simulink model "SoftABS"  (Simulink 7.5)
settings: Solver=ode45  StartTime=0.0  StopTime=inf  RelTol=1e-3
PreLoadFcn:
  | SoftABS_params
undefined symbols (not defined in the file): f_ax, f_slip, sko, sku, T_F_Pres_Free, T_F_Pres_Keep, T_F_Pres_Reduce
libraries: CarMaker4SL x13, simulink x1
(part 1 of 2)
settings Model: Creator=fh  LastModifiedBy=ml  ExtModeAutoUpdateStatusClock=off
settings DataIOCC: SignalLoggingName=sigsOut
settings OptimizationCC: BooleanDataType=off  InitFltsAndDblsToZero=on
settings DebuggingCC: SaveWithParameterizedLinksMsg=none  SignalResolutionControl=TryResolveAllWithWarning  SolverPrmCheckMsg=none  MultiTaskDSMMsg=warning  MultiTaskCondExecSysMsg=none
settings HardwareCC: TargetUnknown=on
settings RTWCC: IncludeERTFirstTime=on
settings CodeAppCC: MaxIdLength=63
settings GRTTargetCC: TargetFcnLib=ansi_tfl_tmw.mat

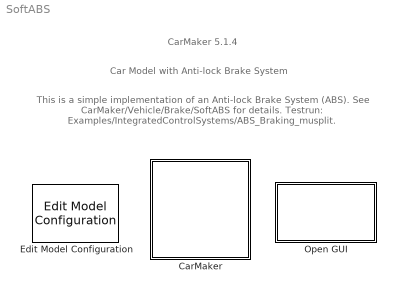
== system SoftABS ==
  note: Car Model with Anti-lock Brake System
  note: CarMaker 5.1.4
  note: This is a simple implementation of an Anti-lock Brake System (ABS).
      | See CarMaker/Vehicle/Brake/SoftABS for details.
      | Testrun: Examples/IntegratedControlSystems/ABS_Braking_musplit.
  CarMaker : Subsystem  TreatAsAtomicUnit=on
      mask Display: image(imread('CarMaker4SLss.bmp'));
  Edit Model Configuration : CarMaker4SL/Edit Model Configuration
  Open GUI : Subsystem  LoadFcn=if ~length(which('cmcmd')), cmenv; end
      settings: OpenFcn=cmblockmagic('gui_fix_display'); CM_Simulink
      mask Display: image(imread('CarMakerGUI.bmp'));

== system SoftABS/CarMaker ==
  CM_FIRST : Subsystem
  CM_LAST : Subsystem
  DrivMan : Subsystem
  Ground : Ground
  Terminator : Terminator
  Vehicle : Subsystem
  VehicleControl : Subsystem
  wires:
  DrivMan/2(DrivMan.Out) -> VehicleControl/2(DrivMan.In)
  DrivMan/1(Sync_Out) -> VehicleControl/1(Sync_In)
  CM_FIRST/2(Env.Misc) -> DrivMan/2(Env.Misc)
  CM_FIRST/1(Sync_Out) -> DrivMan/1(Sync_In)
  CM_LAST/1(Sync_Out) -> Terminator/1
  Ground/1 -> CM_FIRST/1(Sync_In)
  Vehicle/1(Sync_Out) -> CM_LAST/1(Sync_In)
  VehicleControl/1(Sync_Out) -> Vehicle/1(Sync_In)
  VehicleControl/3(VhclCtrl.Steering) -> Vehicle/3(VhclCtrl.Steering)
  VehicleControl/4(Vhcl.Wheel.In) -> Vehicle/4(Vhcl.Wheel.In)
  VehicleControl/5(Vhcl.Misc) -> Vehicle/5(Vhcl.Misc)
  VehicleControl/6(VhclCtrl.Brake) -> Vehicle/6(VhclCtrl.Brake)
  VehicleControl/7(VhclCtrl.PT) -> Vehicle/7(VhclCtrl.PT)
  VehicleControl/2(Vhcl.Model.Source) -> Vehicle/2(Vhcl.Model.Source)

== system SoftABS/Open GUI ==
  S-Function : S-Function  FunctionName=cm_gui  EnableBusSupport=off

== system SoftABS/CarMaker/CM_FIRST ==
  Sync_In : Inport  OutDataType=sfix(16)  OutScaling=2^0
  Bus Creator1 : BusCreator  Inputs=9
  Demux : Demux  Outputs=9
  Environment : S-Function  FunctionName=CM_Sfun  Parameters='Environment'  EnableBusSupport=off
  IoIn : S-Function  FunctionName=CM_Sfun  Parameters='IoIn'  EnableBusSupport=off
  Sync_Out : Outport  OutDataType=sfix(16)  OutScaling=2^0
  Env.Misc : Outport  Port=2  OutDataType=sfix(16)  OutScaling=2^0
  wires:
  Demux/9 -> Bus Creator1/9  "Env WindVel_tot z"
  Demux/8 -> Bus Creator1/8  "Env WindVel_tot y"
  Demux/7 -> Bus Creator1/7  "Env WindVel_tot x"
  Demux/6 -> Bus Creator1/6  "Env SolarRadiation"
  Demux/5 -> Bus Creator1/5  "Env Time"
  Sync_In/1 -> IoIn/1
  IoIn/1 -> Environment/1
  Environment/1 -> Sync_Out/1
  Demux/1 -> Bus Creator1/1  "Env Temperature"
  Demux/2 -> Bus Creator1/2  "Env AirDensity"
  Demux/3 -> Bus Creator1/3  "Env AirPressure"
  Demux/4 -> Bus Creator1/4  "Env AirHumidity"
  Environment/2 -> Demux/1
  Bus Creator1/1 -> Env.Misc/1

== system SoftABS/CarMaker/CM_LAST ==
  Sync_In : Inport  OutDataType=sfix(16)  OutScaling=2^0
  CM_User : S-Function  FunctionName=CM_Sfun  Parameters='CM_User'  EnableBusSupport=off
  IoOut : S-Function  FunctionName=CM_Sfun  Parameters='IoOut'  EnableBusSupport=off
  Sync_Out : Outport  OutDataType=sfix(16)  OutScaling=2^0
  wires:
  IoOut/1 -> Sync_Out/1
  CM_User/1 -> IoOut/1
  Sync_In/1 -> CM_User/1

== system SoftABS/CarMaker/DrivMan ==
  note: There's rarely a reason to override DrivMan signals.
      | Use the VehicleControl interface for this purpose.
  Sync_In : Inport  OutDataType=sfix(16)  OutScaling=2^0
  Env.Misc : Inport  Port=2  OutDataType=sfix(16)  OutScaling=2^0
  BusCreator : BusCreator  Inputs=17
  Demux : Demux  Outputs=17
  DrivMan : S-Function  FunctionName=CM_Sfun  Parameters='DrivMan'  EnableBusSupport=off
  Sync_Out : Outport  OutDataType=sfix(16)  OutScaling=2^0
  DrivMan.Out : Outport  Port=2  OutDataType=sfix(16)  OutScaling=2^0
  wires:
  DrivMan/2 -> Demux/1
  BusCreator/1 -> DrivMan.Out/1
  DrivMan/1 -> Sync_Out/1
  Sync_In/1 -> DrivMan/1
  Env.Misc/1 -> DrivMan/2
  Demux/1 -> BusCreator/1  "DrivMan SST"
  Demux/2 -> BusCreator/2  "DrivMan Key"
  Demux/3 -> BusCreator/3  "DrivMan UserSignal0"
  Demux/4 -> BusCreator/4  "DrivMan UserSignal1"
  Demux/5 -> BusCreator/5  "DrivMan UserSignal2"
  Demux/6 -> BusCreator/6  "DrivMan UserSignal3"
  Demux/7 -> BusCreator/7  "DrivMan UserSignal4"
  Demux/8 -> BusCreator/8  "DrivMan SelectorCtrl"
  Demux/9 -> BusCreator/9  "DrivMan GearNo"
  Demux/10 -> BusCreator/10  "DrivMan Brake"
  Demux/11 -> BusCreator/11  "DrivMan BrakePark"
  Demux/12 -> BusCreator/12  "DrivMan Clutch"
  Demux/13 -> BusCreator/13  "DrivMan Gas"
  Demux/14 -> BusCreator/14  "DrivMan Steering Ang"
  Demux/15 -> BusCreator/15  "DrivMan Steering AngVel"
  Demux/16 -> BusCreator/16  "DrivMan Steering AngAcc"
  Demux/17 -> BusCreator/17  "DrivMan Steering Trq"

== system SoftABS/CarMaker/Vehicle ==
  Sync_In : Inport  OutDataType=sfix(16)  OutScaling=2^0
  Vhcl.Model.Source : Inport  Port=2  OutDataType=sfix(16)  OutScaling=2^0
  VhclCtrl.Steering : Inport  Port=3  OutDataType=sfix(16)  OutScaling=2^0
  Vhcl.Wheel.In : Inport  Port=4  OutDataType=sfix(16)  OutScaling=2^0
  Vhcl.Misc : Inport  Port=5  OutDataType=sfix(16)  OutScaling=2^0
  VhclCtrl.Brake : Inport  Port=6  OutDataType=sfix(16)  OutScaling=2^0
  VhclCtrl.PT : Inport  Port=7  OutDataType=sfix(16)  OutScaling=2^0
  Brake : Subsystem
  CarAndTrailer : Subsystem
  PowerTrain : Subsystem
  Stop Simulation : Stop
  VehicleSource_BuiltIn : simulink/Logic and Bit Operations/Compare To Constant  SystemSampleTime=-1  relop=~=  const=1  LogicOutDataTypeMode=boolean  ZeroCross=off
  Sync_Out : Outport  OutDataType=sfix(16)  OutScaling=2^0
  wires:
  Vhcl.Model.Source/1 -> VehicleSource_BuiltIn/1
  Sync_In/1 -> CarAndTrailer/1(Sync_In)
  VhclCtrl.Steering/1 -> CarAndTrailer/2(VhclCtrl.Steering)
  Vhcl.Wheel.In/1 -> CarAndTrailer/3(Vhcl.Wheel.In)
  Vhcl.Misc/1 -> CarAndTrailer/4(Vhcl.Misc)
  PowerTrain/1(Sync_Out) -> Sync_Out/1
  VhclCtrl.Brake/1 -> Brake/3(VhclCtrl.Brake)
  CarAndTrailer/2(Brake.IF.In) -> Brake/2(Brake.IF.In)
  CarAndTrailer/1(Sync_Out) -> Brake/1(Sync_In)
  VhclCtrl.PT/1 -> PowerTrain/3(VhclCtrl.PT)
  VehicleSource_BuiltIn/1 -> Stop Simulation/1
  Brake/1(Sync_Out) -> PowerTrain/1(Sync_In)
  Brake/2(Vhcl.Wheel.PT) -> PowerTrain/2(Vhcl.Wheel.PT)

== system SoftABS/CarMaker/VehicleControl ==
  note: <Your model here>
  note: When implementing a vehicle control model,
      | be sure to add '-disablevehiclecontrol' to the command line arguments
      | in the CarMaker Model Configuration block.
      | Otherwise your model will possibly not see the original DrivMan signals
      | on its inputs, but those of a currently activated C-coded vehicle control model instead.
  Sync_In : Inport  OutDataType=sfix(16)  OutScaling=2^0
  DrivMan.In : Inport  Port=2  OutDataType=sfix(16)  OutScaling=2^0
  Bus Creator2 : BusCreator  Inputs=2
  CreateBus Vhcl.Misc : Subsystem
  CreateBus Vhcl.Wheel.In : Subsystem
  CreateBus VhclCtrl : Subsystem
  CreateBus VhclCtrl.PT : Subsystem
  CreateBus VhclCtrl.Steering : Subsystem
  Demux2 : Demux  Outputs=2
  VehicleControl : S-Function  FunctionName=CM_Sfun  Parameters='VehicleControl'  EnableBusSupport=off
  VehicleControlUpd : S-Function  FunctionName=CM_Sfun  Parameters='VehicleControlUpd'  EnableBusSupport=off
  Sync_Out : Outport  OutDataType=sfix(16)  OutScaling=2^0
  Vhcl.Model.Source : Outport  Port=2  OutDataType=sfix(16)  OutScaling=2^0
  VhclCtrl.Steering : Outport  Port=3  OutDataType=sfix(16)  OutScaling=2^0
  Vhcl.Wheel.In : Outport  Port=4  OutDataType=sfix(16)  OutScaling=2^0
  Vhcl.Misc : Outport  Port=5  OutDataType=sfix(16)  OutScaling=2^0
  VhclCtrl.Brake : Outport  Port=6  OutDataType=sfix(16)  OutScaling=2^0
  VhclCtrl.PT : Outport  Port=7  OutDataType=sfix(16)  OutScaling=2^0
  wires:
  CreateBus VhclCtrl/1(Out) -> VehicleControlUpd/2
  VehicleControl/2 -> CreateBus VhclCtrl/1(In)
  VehicleControlUpd/2 -> Vhcl.Model.Source/1
  VehicleControlUpd/4 -> CreateBus Vhcl.Wheel.In/1(In1)
  VehicleControlUpd/5 -> CreateBus Vhcl.Misc/1(In1)
  VehicleControlUpd/6 -> Demux2/1
  VehicleControlUpd/7 -> CreateBus VhclCtrl.PT/1(In1)
  VehicleControlUpd/3 -> CreateBus VhclCtrl.Steering/1(In1)
  CreateBus Vhcl.Misc/1(Out1) -> Vhcl.Misc/1
  CreateBus Vhcl.Wheel.In/1(Out1) -> Vhcl.Wheel.In/1
  DrivMan.In/1 -> VehicleControl/2
  VehicleControl/1 -> VehicleControlUpd/1
  Sync_In/1 -> VehicleControl/1
  CreateBus VhclCtrl.PT/1(Out1) -> VhclCtrl.PT/1
  Bus Creator2/1 -> VhclCtrl.Brake/1
  CreateBus VhclCtrl.Steering/1(Out1) -> VhclCtrl.Steering/1
  VehicleControlUpd/1 -> Sync_Out/1
  Demux2/2 -> Bus Creator2/2  "VhclCtrl BrakePark"
  Demux2/1 -> Bus Creator2/1  "VhclCtrl Brake"

== system SoftABS/CarMaker/Vehicle/Brake ==
  note: When replacing the entire braking system,
      | be sure to add '-disablebrake' to the command line arguments
      | in the CarMaker Model Configuration block.
  Sync_In : Inport  OutDataType=sfix(16)  OutScaling=2^0
  Brake.IF.In : Inport  Port=2  OutDataType=sfix(16)  OutScaling=2^0
  VhclCtrl.Brake : Inport  Port=3  OutDataType=sfix(16)  OutScaling=2^0
  Brake : S-Function  FunctionName=CM_Sfun  Parameters='Brake'  EnableBusSupport=off
  BrakeUpd : S-Function  FunctionName=CM_Sfun  Parameters='BrakeUpd'  EnableBusSupport=off
  BusCreator : BusCreator  Inputs=12
  CreateBus Vhcl.Wheel.PT : Subsystem
  Demux : Demux  Outputs=12
  SoftABS : Subsystem
  Sync_Out : Outport  OutDataType=sfix(16)  OutScaling=2^0
  Vhcl.Wheel.PT : Outport  Port=2  OutDataType=sfix(16)  OutScaling=2^0
  wires:
  Brake/1 -> BrakeUpd/1  "Sync"
  Brake.IF.In/1 -> Brake/2
  VhclCtrl.Brake/1 -> Brake/3
  Brake/2 -> Demux/1
  Sync_In/1 -> Brake/1
  BusCreator/1 -> SoftABS/1(Brake.In)
  SoftABS/1(Brake.Out) -> BrakeUpd/2
  Demux/12 -> BusCreator/12  "Brake IF Trq_Reg_trg RR"
  Demux/11 -> BusCreator/11  "Brake IF Trq_Reg_trg RL"
  Demux/10 -> BusCreator/10  "Brake IF Trq_Reg_trg FR"
  Demux/9 -> BusCreator/9  "Brake IF Trq_Reg_trg FL"
  Demux/8 -> BusCreator/8  "Brake IF Trq_PB RR"
  Demux/7 -> BusCreator/7  "Brake IF Trq_PB RL"
  Demux/6 -> BusCreator/6  "Brake IF Trq_PB FR"
  Demux/5 -> BusCreator/5  "Brake IF Trq_PB FL"
  Demux/4 -> BusCreator/4  "Brake IF Trq_WB RR"
  Demux/3 -> BusCreator/3  "Brake IF Trq_WB RL"
  Demux/2 -> BusCreator/2  "Brake IF Trq_WB FR"
  Demux/1 -> BusCreator/1  "Brake IF Trq_WB FL"
  BrakeUpd/1 -> Sync_Out/1
  BrakeUpd/2 -> CreateBus Vhcl.Wheel.PT/1(In)
  CreateBus Vhcl.Wheel.PT/1(Out) -> Vhcl.Wheel.PT/1

== system SoftABS/CarMaker/Vehicle/CarAndTrailer ==
  Sync_In : Inport  OutDataType=sfix(16)  OutScaling=2^0
  VhclCtrl.Steering : Inport  Port=2  OutDataType=sfix(16)  OutScaling=2^0
  Vhcl.Wheel.In : Inport  Port=3  OutDataType=sfix(16)  OutScaling=2^0
  Vhcl.Misc : Inport  Port=4  OutDataType=sfix(16)  OutScaling=2^0
  CarAndTrailerUpd : Subsystem
  Forces : Subsystem
  Ground : Ground
  Kinematics : Subsystem
  Kinetics : Subsystem
  Steering : Subsystem
  Terminator : Terminator
  Terminator1 : Terminator
  Trailer : Subsystem
  Sync_Out : Outport  OutDataType=sfix(16)  OutScaling=2^0
  Brake.IF.In : Outport  Port=2  OutDataType=sfix(16)  OutScaling=2^0
  wires:
  Kinematics/9(lBuf) -> Forces/9(lBuf)
  Forces/12(FBuf) -> Kinetics/12(FBuf)
  Kinematics/8(lStabi) -> Forces/8(lStabi)
  Kinematics/1(Sync_Out) -> Forces/1(Sync_In)
  Kinematics/2(TireFL_In) -> Forces/2(TireFL_In)
  Kinematics/3(TireFR_In) -> Forces/3(TireFR_In)
  Kinematics/4(TireRL_In) -> Forces/4(TireRL_In)
  Kinematics/5(TireRR_In) -> Forces/5(TireRR_In)
  Forces/1(Sync_Out) -> Kinetics/1(Sync_In)
  Forces/3(Car.Aero) -> Kinetics/3(Car.Aero)
  Kinematics/7(vDamp) -> Forces/7(vDamp)
  Kinematics/6(lSpring) -> Forces/6(lSpring)
  Forces/2(Car.Virtual) -> Kinetics/2(Car.Virtual)
  Forces/4(Car.Load) -> Kinetics/4(Car.Load)
  Forces/5(TireFL_Out) -> Kinetics/5(TireFL.Out)
  Forces/6(TireFR_Out) -> Kinetics/6(TireFR.Out)
  Forces/7(TireRL_Out) -> Kinetics/7(TireRL.Out)
  Forces/8(TireRR_Out) -> Kinetics/8(TireRR.Out)
  Forces/9(FSpring) -> Kinetics/9(FSpring)
  Forces/10(FDamp) -> Kinetics/10(FDamp)
  Forces/11(FStabi) -> Kinetics/11(FStabi)
  Ground/1 -> CarAndTrailerUpd/10(Vhcl.Fr1A)
  Kinetics/1(Sync_Out) -> Trailer/1(Sync_In)
  Steering/1(Sync_Out) -> Kinematics/1(Sync_In)
  Sync_In/1 -> Steering/1(Sync_In)
  VhclCtrl.Steering/1 -> Steering/2(VhclCtrl.Steering)
  Kinetics/2(Trailer.Load) -> Trailer/2(Trailer.Load)
  Kinetics/3(Car.Hitch) -> Trailer/3(Car.Hitch)
  Kinetics/4(Car.Fr1) -> Trailer/4(Car.Fr1)
  Steering/2(Steer.IF) -> Kinematics/2(Steer.IF)
  Kinetics/5(Car.Trq_T2W) -> Trailer/5(Car.Trq_T2W)
  Kinetics/6(WheelCarrier.Misc) -> Trailer/6(WheelCarrier.Misc)
  Vhcl.Wheel.In/1 -> Terminator/1
  Vhcl.Misc/1 -> Terminator1/1
  CarAndTrailerUpd/1(Sync_Out) -> Sync_Out/1
  CarAndTrailerUpd/2(Brake.IF.In) -> Brake.IF.In/1
  Trailer/1(Sync_Out) -> CarAndTrailerUpd/1(Sync_In)
  Trailer/2(Vhcl.Steering) -> CarAndTrailerUpd/2(Vhcl.Steering)
  Trailer/3(Vhcl.Motion) -> CarAndTrailerUpd/3(Vhcl.Motion)
  Trailer/4(Vhcl.PoI) -> CarAndTrailerUpd/4(Vhcl.PoI)
  Trailer/5(Vhcl.Wheel.FL) -> CarAndTrailerUpd/5(Vhcl.Wheel.FL)
  Trailer/6(Vhcl.Wheel.FR) -> CarAndTrailerUpd/6(Vhcl.Wheel.FR)
  Trailer/7(Vhcl.Wheel.RL) -> CarAndTrailerUpd/7(Vhcl.Wheel.RL)
  Trailer/8(Vhcl.Wheel.RR) -> CarAndTrailerUpd/8(Vhcl.Wheel.RR)
  Trailer/9(Car.Hitch.FrcTrq) -> CarAndTrailerUpd/9(Car.Hitch.FrcTrq)

== system SoftABS/CarMaker/Vehicle/PowerTrain ==
  note: <Your model here>
  note: When replacing the entire powertrain,
      | be sure to add '-disablepowertrain' to the command line arguments
      | in the CarMaker Model Configuration block.
  Sync_In : Inport  OutDataType=sfix(16)  OutScaling=2^0
  Vhcl.Wheel.PT : Inport  Port=2  OutDataType=sfix(16)  OutScaling=2^0
  VhclCtrl.PT : Inport  Port=3  OutDataType=sfix(16)  OutScaling=2^0
  BusCreator : BusCreator  Inputs=40
  Demux : Demux  Outputs=40
  PowerTrain : S-Function  FunctionName=CM_Sfun  Parameters='PowerTrain'  EnableBusSupport=off
  PowerTrainUpd : S-Function  FunctionName=CM_Sfun  Parameters='PowerTrainUpd'  EnableBusSupport=off
  Sync_Out : Outport  OutDataType=sfix(16)  OutScaling=2^0
  wires:
  Vhcl.Wheel.PT/1 -> PowerTrain/2
  VhclCtrl.PT/1 -> PowerTrain/3
  Demux/40 -> BusCreator/40  "PT IF WRR Trq_BrakeReg_max"
  Demux/39 -> BusCreator/39  "PT IF WRR Trq_BrakeReg"
  Demux/38 -> BusCreator/38  "PT IF WRR Trq_Supp2WC"
  Demux/37 -> BusCreator/37  "PT IF WRR Trq_Drive"
  Demux/36 -> BusCreator/36  "PT IF WRR Trq_B2W"
  Demux/35 -> BusCreator/35  "PT IF WRR rotv"
  Demux/34 -> BusCreator/34  "PT IF WRR rot"
  Demux/33 -> BusCreator/33  "PT IF WRL Trq_BrakeReg_max"
  Demux/32 -> BusCreator/32  "PT IF WRL Trq_BrakeReg"
  Demux/31 -> BusCreator/31  "PT IF WRL Trq_Supp2WC"
  Demux/30 -> BusCreator/30  "PT IF WRL Trq_Drive"
  Demux/29 -> BusCreator/29  "PT IF WRL Trq_B2W"
  Demux/28 -> BusCreator/28  "PT IF WRL rotv"
  Demux/27 -> BusCreator/27  "PT IF WRL rot"
  Demux/26 -> BusCreator/26  "PT IF WFR Trq_BrakeReg_max"
  Demux/25 -> BusCreator/25  "PT IF WFR Trq_BrakeReg"
  Demux/24 -> BusCreator/24  "PT IF WFR Trq_Supp2WC"
  Demux/23 -> BusCreator/23  "PT IF WFR Trq_Drive"
  Demux/22 -> BusCreator/22  "PT IF WFR Trq_B2W"
  Demux/21 -> BusCreator/21  "PT IF WFR rotv"
  Demux/20 -> BusCreator/20  "PT IF WFR rot"
  Demux/19 -> BusCreator/19  "PT IF WFL Trq_BrakeReg_max"
  Demux/18 -> BusCreator/18  "PT IF WFL Trq_BrakeReg"
  Demux/17 -> BusCreator/17  "PT IF WFL Trq_Supp2WC"
  Demux/16 -> BusCreator/16  "PT IF WFL Trq_Drive"
  Demux/15 -> BusCreator/15  "PT IF WFL Trq_B2W"
  Demux/14 -> BusCreator/14  "PT IF WFL rotv"
  Demux/13 -> BusCreator/13  "PT IF WFL rot"
  Demux/12 -> BusCreator/12  "PT IF DL_iDiff_mean"
  Demux/11 -> BusCreator/11  "PT IF Trq_Supp2BdyEng y"
  Demux/10 -> BusCreator/10  "PT IF Trq_Supp2BdyEng x"
  Demux/9 -> BusCreator/9  "PT IF Trq_Supp2Bdy1 z"
  Demux/8 -> BusCreator/8  "PT IF Trq_Supp2Bdy1 y"
  Demux/7 -> BusCreator/7  "PT IF Trq_Supp2Bdy1 x"
  Demux/6 -> BusCreator/6  "PT IF Engine_Trq (EngineControl)"
  Demux/5 -> BusCreator/5  "PT IF Engine_rotv"
  Demux/4 -> BusCreator/4  "PT IF GearNo"
  Demux/3 -> BusCreator/3  "PT IF OperationError"
  Demux/2 -> BusCreator/2  "PT IF OperationState"
  Demux/1 -> BusCreator/1  "PT IF Ignition"
  BusCreator/1 -> PowerTrainUpd/2
  PowerTrain/1 -> PowerTrainUpd/1  "Sync"
  PowerTrainUpd/1 -> Sync_Out/1
  PowerTrain/2 -> Demux/1
  Sync_In/1 -> PowerTrain/1

== system SoftABS/CarMaker/VehicleControl/CreateBus Vhcl.Misc ==
  In1 : Inport  OutDataType=sfix(16)  OutScaling=2^0
  Bus Creator5 : BusCreator  Inputs=11
  Demux5 : Demux  Outputs=11
  Out1 : Outport  OutDataType=sfix(16)  OutScaling=2^0
  wires:
  Demux5/11 -> Bus Creator5/11  "Vhcl Wind_vel_0 z"
  Demux5/10 -> Bus Creator5/10  "Vhcl Wind_vel_0 y"
  Demux5/9 -> Bus Creator5/9  "Vhcl Wind_vel_0 x"
  Demux5/8 -> Bus Creator5/8  "Vhcl DL2BdyEng y"
  Demux5/7 -> Bus Creator5/7  "Vhcl DL2BdyEng x"
  Demux5/6 -> Bus Creator5/6  "Vhcl TrqDL2Bdy1B z"
  Demux5/5 -> Bus Creator5/5  "Vhcl TrqDL2Bdy1B y"
  Demux5/4 -> Bus Creator5/4  "Vhcl TrqDL2Bdy1B x"
  Demux5/3 -> Bus Creator5/3  "Vhcl Trq_DL2Bdy1 z"
  In1/1 -> Demux5/1
  Bus Creator5/1 -> Out1/1
  Demux5/2 -> Bus Creator5/2  "Vhcl Trq_DL2Bdy1 y"
  Demux5/1 -> Bus Creator5/1  "Vhcl Trq_DL2Bdy1 x"

== system SoftABS/CarMaker/VehicleControl/CreateBus Vhcl.Wheel.In ==
  In1 : Inport  OutDataType=sfix(16)  OutScaling=2^0
  Bus Creator1 : BusCreator  Inputs=12
  Demux1 : Demux  Outputs=12
  Out1 : Outport  OutDataType=sfix(16)  OutScaling=2^0
  wires:
  Demux1/12 -> Bus Creator1/12  "Vhcl Wheel RR rotv"
  Demux1/11 -> Bus Creator1/11  "Vhcl Wheel RR Trq_DL2WC"
  Demux1/10 -> Bus Creator1/10  "Vhcl Wheel RR Trq_B2WC"
  Demux1/9 -> Bus Creator1/9  "Vhcl Wheel RL rotv"
  Demux1/8 -> Bus Creator1/8  "Vhcl Wheel RL Trq_DL2WC"
  Demux1/7 -> Bus Creator1/7  "Vhcl Wheel RL Trq_B2WC"
  Demux1/6 -> Bus Creator1/6  "Vhcl Wheel FR rotv"
  Demux1/5 -> Bus Creator1/5  "Vhcl Wheel FR Trq_DL2WC"
  Demux1/4 -> Bus Creator1/4  "Vhcl Wheel FR Trq_B2WC"
  Demux1/3 -> Bus Creator1/3  "Vhcl Wheel FL rotv"
  In1/1 -> Demux1/1
  Bus Creator1/1 -> Out1/1
  Demux1/2 -> Bus Creator1/2  "Vhcl Wheel FL Trq_DL2WC"
  Demux1/1 -> Bus Creator1/1  "Vhcl Wheel FL Trq_B2WC"

== system SoftABS/CarMaker/VehicleControl/CreateBus VhclCtrl ==
  In : Inport
  BusCreator : BusCreator  Inputs=29
  Demux : Demux  Outputs=29
  Out : Outport
  wires:
  In/1 -> Demux/1
  BusCreator/1 -> Out/1
  Demux/1 -> BusCreator/1  "VhclCtrl SST"
  Demux/2 -> BusCreator/2  "VhclCtrl Key"
  Demux/3 -> BusCreator/3  "VhclCtrl UserSignal0"
  Demux/4 -> BusCreator/4  "VhclCtrl UserSignal1"
  Demux/5 -> BusCreator/5  "VhclCtrl UserSignal2"
  Demux/6 -> BusCreator/6  "VhclCtrl UserSignal3"
  Demux/7 -> BusCreator/7  "VhclCtrl UserSignal4"
  Demux/8 -> BusCreator/8  "VhclCtrl GearNo"
  Demux/9 -> BusCreator/9  "VhclCtrl SelectorCtrl"
  Demux/10 -> BusCreator/10  "VhclCtrl Brake"
  Demux/11 -> BusCreator/11  "VhclCtrl BrakePark"
  Demux/12 -> BusCreator/12  "VhclCtrl Clutch"
  Demux/13 -> BusCreator/13  "VhclCtrl Gas"
  Demux/14 -> BusCreator/14  "VhclCtrl Steering Ang"
  Demux/15 -> BusCreator/15  "VhclCtrl Steering AngVel"
  Demux/16 -> BusCreator/16  "VhclCtrl Steering AngAcc"
  Demux/17 -> BusCreator/17  "VhclCtrl Steering Trq"
  Demux/18 -> BusCreator/18  "VhclCtrl Lights LowBeam"
  Demux/19 -> BusCreator/19  "VhclCtrl Lights HighBeam"
  Demux/20 -> BusCreator/20  "VhclCtrl Lights Daytime"
  Demux/21 -> BusCreator/21  "VhclCtrl Lights ParkL"
  Demux/22 -> BusCreator/22  "VhclCtrl Lights ParkR"
  Demux/23 -> BusCreator/23  "VhclCtrl Lights IndL"
  Demux/24 -> BusCreator/24  "VhclCtrl Lights IndR"
  Demux/25 -> BusCreator/25  "VhclCtrl Lights FogFrontL"
  Demux/26 -> BusCreator/26  "VhclCtrl Lights FogFrontR"
  Demux/27 -> BusCreator/27  "VhclCtrl Lights FogRear"
  Demux/28 -> BusCreator/28  "VhclCtrl Lights Brake"
  Demux/29 -> BusCreator/29  "VhclCtrl Lights Reverse"

== system SoftABS/CarMaker/VehicleControl/CreateBus VhclCtrl.PT ==
  In1 : Inport
  BusCreator : BusCreator  Inputs=11
  Demux : Demux  Outputs=11
  Out1 : Outport
  wires:
  In1/1 -> Demux/1
  BusCreator/1 -> Out1/1
  Demux/1 -> BusCreator/1  "VhclCtrl SST"
  Demux/2 -> BusCreator/2  "VhclCtrl Key"
  Demux/3 -> BusCreator/3  "VhclCtrl UserSignal0"
  Demux/4 -> BusCreator/4  "VhclCtrl UserSignal1"
  Demux/5 -> BusCreator/5  "VhclCtrl UserSignal2"
  Demux/6 -> BusCreator/6  "VhclCtrl UserSignal3"
  Demux/7 -> BusCreator/7  "VhclCtrl UserSignal4"
  Demux/8 -> BusCreator/8  "VhclCtrl GearNo"
  Demux/9 -> BusCreator/9  "VhclCtrl SelectorCtrl"
  Demux/10 -> BusCreator/10  "VhclCtrl Clutch"
  Demux/11 -> BusCreator/11  "VhclCtrl Gas"

== system SoftABS/CarMaker/VehicleControl/CreateBus VhclCtrl.Steering ==
  In1 : Inport  OutDataType=sfix(16)  OutScaling=2^0
  Bus Creator : BusCreator  Inputs=5
  Demux : Demux  Outputs=5
  Out1 : Outport  OutDataType=sfix(16)  OutScaling=2^0
  wires:
  In1/1 -> Demux/1
  Bus Creator/1 -> Out1/1
  Demux/1 -> Bus Creator/1  "VhclCtrl Steering Ang"
  Demux/5 -> Bus Creator/5  "VhclCtrl Steering ByTrq"
  Demux/3 -> Bus Creator/3  "VhclCtrl Steering AngAcc"
  Demux/2 -> Bus Creator/2  "VhclCtrl Steering AngVel"
  Demux/4 -> Bus Creator/4  "VhclCtrl Steering Trq"

== system SoftABS/CarMaker/Vehicle/Brake/CreateBus Vhcl.Wheel.PT ==
  In : Inport
  BusCreator : BusCreator  Inputs=16
  Demux : Demux  Outputs=16
  Out : Outport
  wires:
  In/1 -> Demux/1
  BusCreator/1 -> Out/1
  Demux/1 -> BusCreator/1  "Vhcl Wheel FL Trq_Brake"
  Demux/2 -> BusCreator/2  "Vhcl Wheel FL Trq_BrakeReg_trg"
  Demux/3 -> BusCreator/3  "Vhcl Wheel FL Trq_T2W"
  Demux/4 -> BusCreator/4  "Vhcl Wheel FL WhlBearing"
  Demux/5 -> BusCreator/5  "Vhcl Wheel FR Trq_Brake"
  Demux/6 -> BusCreator/6  "Vhcl Wheel FR Trq_BrakeReg_trg"
  Demux/7 -> BusCreator/7  "Vhcl Wheel FR Trq_T2W"
  Demux/8 -> BusCreator/8  "Vhcl Wheel FR WhlBearing"
  Demux/9 -> BusCreator/9  "Vhcl Wheel RL Trq_Brake"
  Demux/10 -> BusCreator/10  "Vhcl Wheel RL Trq_BrakeReg_trg"
  Demux/11 -> BusCreator/11  "Vhcl Wheel RL Trq_T2W"
  Demux/12 -> BusCreator/12  "Vhcl Wheel RL WhlBearing"
  Demux/13 -> BusCreator/13  "Vhcl Wheel RR Trq_Brake"
  Demux/14 -> BusCreator/14  "Vhcl Wheel RR Trq_BrakeReg_trg"
  Demux/15 -> BusCreator/15  "Vhcl Wheel RR Trq_T2W"
  Demux/16 -> BusCreator/16  "Vhcl Wheel RR WhlBearing"

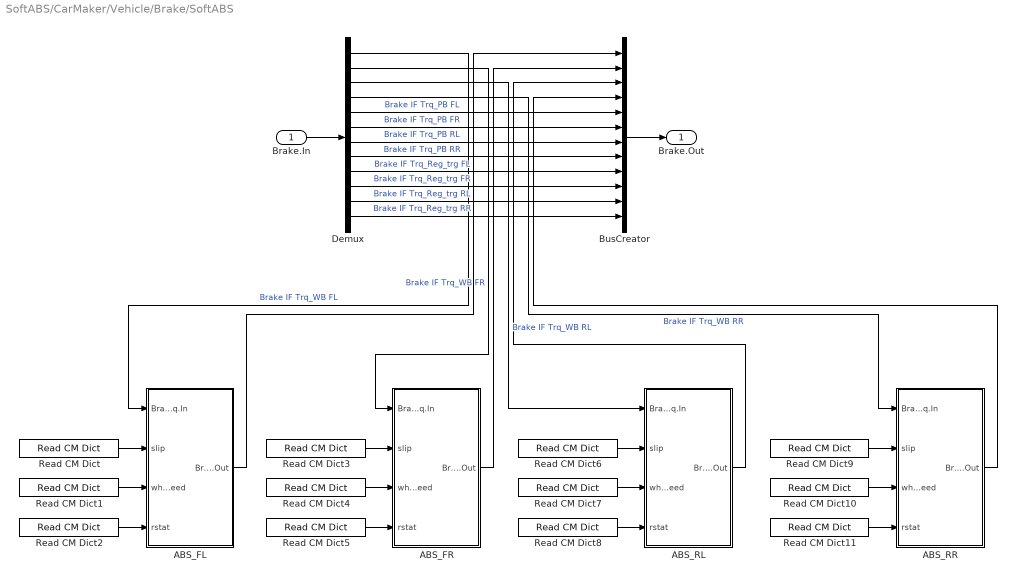
== system SoftABS/CarMaker/Vehicle/Brake/SoftABS ==
  Brake.In : Inport  OutDataType=sfix(16)  OutScaling=2^0
  ABS_FL : Subsystem
  ABS_FR : Subsystem
  ABS_RL : Subsystem
  ABS_RR : Subsystem
  BusCreator : BusCreator  Inputs=12
  Demux : Demux  Outputs=12
  Read CM Dict : CarMaker4SL/Read CM Dict  xname=Car.LongSlipFL  xsync=off
  Read CM Dict1 : CarMaker4SL/Read CM Dict  xname=Car.WheelSpd_FL  xsync=off
  Read CM Dict10 : CarMaker4SL/Read CM Dict  xname=Car.WheelSpd_RR  xsync=off
  Read CM Dict11 : CarMaker4SL/Read CM Dict  xname=Car.WRR.Radius  xsync=off
  Read CM Dict2 : CarMaker4SL/Read CM Dict  xname=Car.WFL.Radius  xsync=off
  Read CM Dict3 : CarMaker4SL/Read CM Dict  xname=Car.LongSlipFR  xsync=off
  Read CM Dict4 : CarMaker4SL/Read CM Dict  xname=Car.WheelSpd_FR  xsync=off
  Read CM Dict5 : CarMaker4SL/Read CM Dict  xname=Car.WFR.Radius  xsync=off
  Read CM Dict6 : CarMaker4SL/Read CM Dict  xname=Car.LongSlipRL  xsync=off
  Read CM Dict7 : CarMaker4SL/Read CM Dict  xname=Car.WheelSpd_RL  xsync=off
  Read CM Dict8 : CarMaker4SL/Read CM Dict  xname=Car.WRL.Radius  xsync=off
  Read CM Dict9 : CarMaker4SL/Read CM Dict  xname=Car.LongSlipRR  xsync=off
  Brake.Out : Outport  OutDataType=sfix(16)  OutScaling=2^0
  wires:
  BusCreator/1 -> Brake.Out/1
  Read CM Dict11/1 -> ABS_RR/4(rstat)
  Read CM Dict10/1 -> ABS_RR/3(wheelspeed)
  Read CM Dict9/1 -> ABS_RR/2(slip)
  Read CM Dict8/1 -> ABS_RL/4(rstat)
  Read CM Dict7/1 -> ABS_RL/3(wheelspeed)
  Read CM Dict6/1 -> ABS_RL/2(slip)
  Read CM Dict5/1 -> ABS_FR/4(rstat)
  Read CM Dict4/1 -> ABS_FR/3(wheelspeed)
  Read CM Dict3/1 -> ABS_FR/2(slip)
  Read CM Dict2/1 -> ABS_FL/4(rstat)
  Read CM Dict1/1 -> ABS_FL/3(wheelspeed)
  Read CM Dict/1 -> ABS_FL/2(slip)
  Brake.In/1 -> Demux/1
  Demux/12 -> BusCreator/12  "Brake IF Trq_Reg_trg RR"
  Demux/11 -> BusCreator/11  "Brake IF Trq_Reg_trg RL"
  Demux/10 -> BusCreator/10  "Brake IF Trq_Reg_trg FR"
  Demux/9 -> BusCreator/9  "Brake IF Trq_Reg_trg FL"
  Demux/8 -> BusCreator/8  "Brake IF Trq_PB RR"
  Demux/7 -> BusCreator/7  "Brake IF Trq_PB RL"
  Demux/6 -> BusCreator/6  "Brake IF Trq_PB FR"
  Demux/5 -> BusCreator/5  "Brake IF Trq_PB FL"
  Demux/1 -> ABS_FL/1(Brake.Trq.In)  "Brake IF Trq_WB FL"
  Demux/2 -> ABS_FR/1(Brake.Trq.In)  "Brake IF Trq_WB FR"
  ABS_FL/1(Brake.Trq.Out) -> BusCreator/1
  ABS_FR/1(Brake.Trq.Out) -> BusCreator/2
  Demux/3 -> ABS_RL/1(Brake.Trq.In)  "Brake IF Trq_WB RL"
  Demux/4 -> ABS_RR/1(Brake.Trq.In)  "Brake IF Trq_WB RR"
  ABS_RR/1(Brake.Trq.Out) -> BusCreator/4
  ABS_RL/1(Brake.Trq.Out) -> BusCreator/3

== system SoftABS/CarMaker/Vehicle/CarAndTrailer/CarAndTrailerUpd ==
  Sync_In : Inport  OutDataType=sfix(16)  OutScaling=2^0
  Vhcl.Steering : Inport  Port=2  OutDataType=sfix(16)  OutScaling=2^0
  Vhcl.Motion : Inport  Port=3  OutDataType=sfix(16)  OutScaling=2^0
  Vhcl.PoI : Inport  Port=4  OutDataType=sfix(16)  OutScaling=2^0
  Vhcl.Wheel.FL : Inport  Port=5  OutDataType=sfix(16)  OutScaling=2^0
  Vhcl.Wheel.FR : Inport  Port=6  OutDataType=sfix(16)  OutScaling=2^0
  Vhcl.Wheel.RL : Inport  Port=7  OutDataType=sfix(16)  OutScaling=2^0
  Vhcl.Wheel.RR : Inport  Port=8  OutDataType=sfix(16)  OutScaling=2^0
  Car.Hitch.FrcTrq : Inport  Port=9  OutDataType=sfix(16)  OutScaling=2^0
  Vhcl.Fr1A : Inport  Port=10  OutDataType=sfix(16)  OutScaling=2^0
  CarAndTrailerUpd : S-Function  FunctionName=CM_Sfun  Parameters='CarAndTrUpd'  EnableBusSupport=off
  CreateBus Brake.IF.In : Subsystem
  Sync_Out : Outport  OutDataType=sfix(16)  OutScaling=2^0
  Brake.IF.In : Outport  Port=2  OutDataType=sfix(16)  OutScaling=2^0
  wires:
  Sync_In/1 -> CarAndTrailerUpd/1
  CarAndTrailerUpd/1 -> Sync_Out/1
  CreateBus Brake.IF.In/1(Out) -> Brake.IF.In/1
  CarAndTrailerUpd/2 -> CreateBus Brake.IF.In/1(In)
  Vhcl.Wheel.RL/1 -> CarAndTrailerUpd/7
  Vhcl.Wheel.RR/1 -> CarAndTrailerUpd/8
  Car.Hitch.FrcTrq/1 -> CarAndTrailerUpd/9
  Vhcl.Wheel.FR/1 -> CarAndTrailerUpd/6
  Vhcl.Wheel.FL/1 -> CarAndTrailerUpd/5
  Vhcl.PoI/1 -> CarAndTrailerUpd/4
  Vhcl.Motion/1 -> CarAndTrailerUpd/3
  Vhcl.Steering/1 -> CarAndTrailerUpd/2
  Vhcl.Fr1A/1 -> CarAndTrailerUpd/10  "user vehicle only"

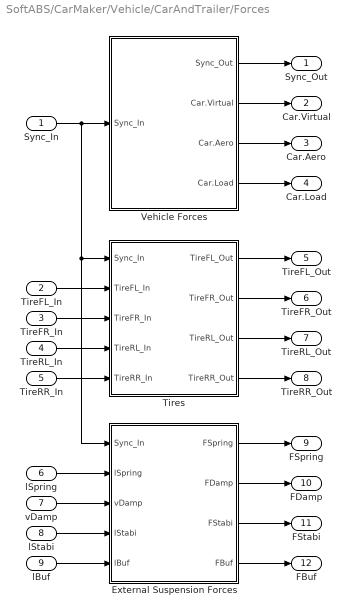
== system SoftABS/CarMaker/Vehicle/CarAndTrailer/Forces ==
  Sync_In : Inport  OutDataType=sfix(16)  OutScaling=2^0
  TireFL_In : Inport  Port=2  OutDataType=sfix(16)  OutScaling=2^0
  TireFR_In : Inport  Port=3  OutDataType=sfix(16)  OutScaling=2^0
  TireRL_In : Inport  Port=4  OutDataType=sfix(16)  OutScaling=2^0
  TireRR_In : Inport  Port=5  OutDataType=sfix(16)  OutScaling=2^0
  lSpring : Inport  Port=6  OutDataType=sfix(16)  OutScaling=2^0
  vDamp : Inport  Port=7  OutDataType=sfix(16)  OutScaling=2^0
  lStabi : Inport  Port=8  OutDataType=sfix(16)  OutScaling=2^0
  lBuf : Inport  Port=9  OutDataType=sfix(16)  OutScaling=2^0
  External Suspension Forces : Subsystem
  Tires : Subsystem
  Vehicle Forces : Subsystem
  Sync_Out : Outport  OutDataType=sfix(16)  OutScaling=2^0
  Car.Virtual : Outport  Port=2  OutDataType=sfix(16)  OutScaling=2^0
  Car.Aero : Outport  Port=3  OutDataType=sfix(16)  OutScaling=2^0
  Car.Load : Outport  Port=4  OutDataType=sfix(16)  OutScaling=2^0
  TireFL_Out : Outport  Port=5  OutDataType=sfix(16)  OutScaling=2^0
  TireFR_Out : Outport  Port=6  OutDataType=sfix(16)  OutScaling=2^0
  TireRL_Out : Outport  Port=7  OutDataType=sfix(16)  OutScaling=2^0
  TireRR_Out : Outport  Port=8  OutDataType=sfix(16)  OutScaling=2^0
  FSpring : Outport  Port=9  OutDataType=sfix(16)  OutScaling=2^0
  FDamp : Outport  Port=10  OutDataType=sfix(16)  OutScaling=2^0
  FStabi : Outport  Port=11  OutDataType=sfix(16)  OutScaling=2^0
  FBuf : Outport  Port=12  OutDataType=sfix(16)  OutScaling=2^0
  wires:
  External Suspension Forces/1(FSpring) -> FSpring/1
  External Suspension Forces/3(FStabi) -> FStabi/1
  lStabi/1 -> External Suspension Forces/4(lStabi)
  vDamp/1 -> External Suspension Forces/3(vDamp)
  External Suspension Forces/2(FDamp) -> FDamp/1
  lSpring/1 -> External Suspension Forces/2(lSpring)
  Vehicle Forces/4(Car.Load) -> Car.Load/1
  Vehicle Forces/3(Car.Aero) -> Car.Aero/1
  Vehicle Forces/2(Car.Virtual) -> Car.Virtual/1
  TireFL_In/1 -> Tires/2(TireFL_In)
  Vehicle Forces/1(Sync_Out) -> Sync_Out/1
  Sync_In/1 -> Vehicle Forces/1(Sync_In), External Suspension Forces/1(Sync_In), Tires/1(Sync_In)
  TireFR_In/1 -> Tires/3(TireFR_In)
  TireRL_In/1 -> Tires/4(TireRL_In)
  TireRR_In/1 -> Tires/5(TireRR_In)
  Tires/1(TireFL_Out) -> TireFL_Out/1
  Tires/2(TireFR_Out) -> TireFR_Out/1
  Tires/3(TireRL_Out) -> TireRL_Out/1
  Tires/4(TireRR_Out) -> TireRR_Out/1
  lBuf/1 -> External Suspension Forces/5(lBuf)
  External Suspension Forces/4(FBuf) -> FBuf/1

== system SoftABS/CarMaker/Vehicle/CarAndTrailer/Kinematics ==
  Sync_In : Inport  OutDataType=sfix(16)  OutScaling=2^0
  Steer.IF : Inport  Port=2  OutDataType=sfix(16)  OutScaling=2^0
  Kinematics : S-Function  FunctionName=CM_Sfun  Parameters='Kinematics'  EnableBusSupport=off
  Sync_Out : Outport  OutDataType=sfix(16)  OutScaling=2^0
  TireFL_In : Outport  Port=2  OutDataType=sfix(16)  OutScaling=2^0
  TireFR_In : Outport  Port=3  OutDataType=sfix(16)  OutScaling=2^0
  TireRL_In : Outport  Port=4  OutDataType=sfix(16)  OutScaling=2^0
  TireRR_In : Outport  Port=5  OutDataType=sfix(16)  OutScaling=2^0
  lSpring : Outport  Port=6  OutDataType=sfix(16)  OutScaling=2^0
  vDamp : Outport  Port=7  OutDataType=sfix(16)  OutScaling=2^0
  lStabi : Outport  Port=8  OutDataType=sfix(16)  OutScaling=2^0
  lBuf : Outport  Port=9  OutDataType=sfix(16)  OutScaling=2^0
  wires:
  Steer.IF/1 -> Kinematics/2
  Kinematics/1 -> Sync_Out/1
  Sync_In/1 -> Kinematics/1
  Kinematics/7 -> vDamp/1
  Kinematics/6 -> lSpring/1
  Kinematics/5 -> TireRR_In/1
  Kinematics/4 -> TireRL_In/1
  Kinematics/3 -> TireFR_In/1
  Kinematics/2 -> TireFL_In/1
  Kinematics/8 -> lStabi/1
  Kinematics/9 -> lBuf/1

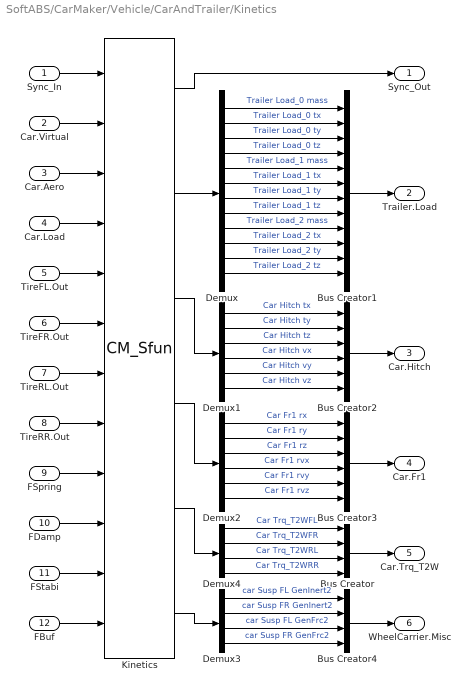
== system SoftABS/CarMaker/Vehicle/CarAndTrailer/Kinetics ==
  Sync_In : Inport  OutDataType=sfix(16)  OutScaling=2^0
  Car.Virtual : Inport  Port=2  OutDataType=sfix(16)  OutScaling=2^0
  Car.Aero : Inport  Port=3  OutDataType=sfix(16)  OutScaling=2^0
  Car.Load : Inport  Port=4  OutDataType=sfix(16)  OutScaling=2^0
  TireFL.Out : Inport  Port=5  OutDataType=sfix(16)  OutScaling=2^0
  TireFR.Out : Inport  Port=6  OutDataType=sfix(16)  OutScaling=2^0
  TireRL.Out : Inport  Port=7  OutDataType=sfix(16)  OutScaling=2^0
  TireRR.Out : Inport  Port=8  OutDataType=sfix(16)  OutScaling=2^0
  FSpring : Inport  Port=9  OutDataType=sfix(16)  OutScaling=2^0
  FDamp : Inport  Port=10  OutDataType=sfix(16)  OutScaling=2^0
  FStabi : Inport  Port=11  OutDataType=sfix(16)  OutScaling=2^0
  FBuf : Inport  Port=12  OutDataType=sfix(16)  OutScaling=2^0
  Bus Creator : BusCreator
  Bus Creator1 : BusCreator  Inputs=12
  Bus Creator2 : BusCreator  Inputs=6
  Bus Creator3 : BusCreator  Inputs=6
  Bus Creator4 : BusCreator
  Demux : Demux  Outputs=12
  Demux1 : Demux  Outputs=6
  Demux2 : Demux  Outputs=6
  Demux3 : Demux
  Demux4 : Demux
  Kinetics : S-Function  FunctionName=CM_Sfun  Parameters='Kinetics'  EnableBusSupport=off
  Sync_Out : Outport  OutDataType=sfix(16)  OutScaling=2^0
  Trailer.Load : Outport  Port=2  OutDataType=sfix(16)  OutScaling=2^0
  Car.Hitch : Outport  Port=3  OutDataType=sfix(16)  OutScaling=2^0
  Car.Fr1 : Outport  Port=4  OutDataType=sfix(16)  OutScaling=2^0
  Car.Trq_T2W : Outport  Port=5  OutDataType=sfix(16)  OutScaling=2^0
  WheelCarrier.Misc : Outport  Port=6  OutDataType=sfix(16)  OutScaling=2^0
  wires:
  Kinetics/5 -> Demux4/1
  Kinetics/6 -> Demux3/1
  FStabi/1 -> Kinetics/11
  FDamp/1 -> Kinetics/10
  FSpring/1 -> Kinetics/9
  TireRR.Out/1 -> Kinetics/8
  TireRL.Out/1 -> Kinetics/7
  TireFR.Out/1 -> Kinetics/6
  TireFL.Out/1 -> Kinetics/5
  Demux4/1 -> Bus Creator/1  "Car Trq_T2WFL"
  Demux4/2 -> Bus Creator/2  "Car Trq_T2WFR"
  Demux4/3 -> Bus Creator/3  "Car Trq_T2WRL"
  Demux4/4 -> Bus Creator/4  "Car Trq_T2WRR"
  Bus Creator/1 -> Car.Trq_T2W/1
  Bus Creator4/1 -> WheelCarrier.Misc/1
  Demux3/4 -> Bus Creator4/4  "car Susp FR GenFrc2"
  Demux3/3 -> Bus Creator4/3  "car Susp FL GenFrc2"
  Demux3/2 -> Bus Creator4/2  "car Susp FR GenInert2"
  Demux3/1 -> Bus Creator4/1  "car Susp FL GenInert2"
  Car.Load/1 -> Kinetics/4
  Kinetics/4 -> Demux2/1
  Bus Creator3/1 -> Car.Fr1/1
  Demux2/6 -> Bus Creator3/6  "Car Fr1 rvz"
  Demux2/5 -> Bus Creator3/5  "Car Fr1 rvy"
  Demux2/4 -> Bus Creator3/4  "Car Fr1 rvx"
  Demux2/3 -> Bus Creator3/3  "Car Fr1 rz"
  Demux2/2 -> Bus Creator3/2  "Car Fr1 ry"
  Demux2/1 -> Bus Creator3/1  "Car Fr1 rx"
  Bus Creator2/1 -> Car.Hitch/1
  Kinetics/3 -> Demux1/1
  Demux1/6 -> Bus Creator2/6  "Car Hitch vz"
  Demux1/5 -> Bus Creator2/5  "Car Hitch vy"
  Demux1/4 -> Bus Creator2/4  "Car Hitch vx"
  Demux1/3 -> Bus Creator2/3  "Car Hitch tz"
  Demux1/2 -> Bus Creator2/2  "Car Hitch ty"
  Demux1/1 -> Bus Creator2/1  "Car Hitch tx"
  Demux/12 -> Bus Creator1/12  "Trailer Load_2 tz"
  Demux/11 -> Bus Creator1/11  "Trailer Load_2 ty"
  Demux/10 -> Bus Creator1/10  "Trailer Load_2 tx"
  Demux/9 -> Bus Creator1/9  "Trailer Load_2 mass"
  Demux/8 -> Bus Creator1/8  "Trailer Load_1 tz"
  Demux/7 -> Bus Creator1/7  "Trailer Load_1 ty"
  Demux/6 -> Bus Creator1/6  "Trailer Load_1 tx"
  Demux/5 -> Bus Creator1/5  "Trailer Load_1 mass"
  Kinetics/2 -> Demux/1
  Demux/4 -> Bus Creator1/4  "Trailer Load_0 tz"
  Demux/3 -> Bus Creator1/3  "Trailer Load_0 ty"
  Demux/2 -> Bus Creator1/2  "Trailer Load_0 tx"
  Demux/1 -> Bus Creator1/1  "Trailer Load_0 mass"
  Bus Creator1/1 -> Trailer.Load/1
  Car.Virtual/1 -> Kinetics/2
  Car.Aero/1 -> Kinetics/3
  Kinetics/1 -> Sync_Out/1
  Sync_In/1 -> Kinetics/1
  FBuf/1 -> Kinetics/12

== system SoftABS/CarMaker/Vehicle/CarAndTrailer/Steering ==
  note: When replacing the entire steering system,
      | be sure to add '-disablesteering' to the command line arguments
      | in the CarMaker Model Configuration block.
  Sync_In : Inport  OutDataType=sfix(16)  OutScaling=2^0
  VhclCtrl.Steering : Inport  Port=2  OutDataType=sfix(16)  OutScaling=2^0
  Bus Creator1 : BusCreator  Inputs=16
  Bus Creator2 : BusCreator
  Demux : Demux  Outputs=20
  Steering : S-Function  FunctionName=CM_Sfun  Parameters='Steering'  EnableBusSupport=off
  Terminator : Terminator
  Sync_Out : Outport  OutDataType=sfix(16)  OutScaling=2^0
  Steer.IF : Outport  Port=2  OutDataType=sfix(16)  OutScaling=2^0
  wires:
  Demux/5 -> Bus Creator1/5  "Steering IF TrqStatic"
  Demux/4 -> Bus Creator1/4  "Steering IF Trq"
  Demux/3 -> Bus Creator1/3  "Steering IF AngAcc"
  Demux/2 -> Bus Creator1/2  "Steering IF AngVel"
  Demux/1 -> Bus Creator1/1  "Steering IF Ang"
  Sync_In/1 -> Steering/1
  Steering/1 -> Sync_Out/1
  VhclCtrl.Steering/1 -> Steering/2
  Demux/15 -> Bus Creator1/15  "Steering IF R qpp"
  Demux/14 -> Bus Creator1/14  "Steering IF R qp"
  Demux/13 -> Bus Creator1/13  "Steering IF R q"
  Demux/12 -> Bus Creator1/12  "Steering IF L iSteer2q"
  Demux/11 -> Bus Creator1/11  "Steering IF L qpp"
  Demux/10 -> Bus Creator1/10  "Steering IF L qp"
  Demux/9 -> Bus Creator1/9  "Steering IF L q"
  Demux/16 -> Bus Creator1/16  "Steering IF R iSteer2q"
  Bus Creator2/1 -> Terminator/1  "Steer IF (in)"
  Demux/19 -> Bus Creator2/3  "Steering IF R Frc"
  Demux/18 -> Bus Creator2/2  "Steering IF L Inert"
  Demux/17 -> Bus Creator2/1  "Steering IF L Frc"
  Demux/20 -> Bus Creator2/4  "Steering IF R Inert"
  Demux/6 -> Bus Creator1/6  "Steering IF AssistFrc"
  Demux/7 -> Bus Creator1/7  "Steering IF AssistTrqCol"
  Demux/8 -> Bus Creator1/8  "Steering IF AssistTrqPin"
  Steering/2 -> Demux/1
  Bus Creator1/1 -> Steer.IF/1

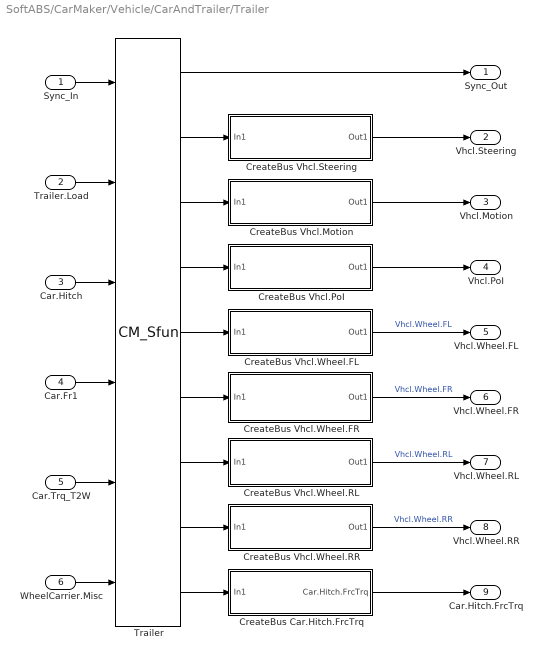
== system SoftABS/CarMaker/Vehicle/CarAndTrailer/Trailer ==
  Sync_In : Inport  OutDataType=sfix(16)  OutScaling=2^0
  Trailer.Load : Inport  Port=2  OutDataType=sfix(16)  OutScaling=2^0
  Car.Hitch : Inport  Port=3  OutDataType=sfix(16)  OutScaling=2^0
  Car.Fr1 : Inport  Port=4  OutDataType=sfix(16)  OutScaling=2^0
  Car.Trq_T2W : Inport  Port=5  OutDataType=sfix(16)  OutScaling=2^0
  WheelCarrier.Misc : Inport  Port=6  OutDataType=sfix(16)  OutScaling=2^0
  CreateBus Car.Hitch.FrcTrq : Subsystem
  CreateBus Vhcl.Motion : Subsystem
  CreateBus Vhcl.PoI : Subsystem
  CreateBus Vhcl.Steering : Subsystem
  CreateBus Vhcl.Wheel.FL : Subsystem
  CreateBus Vhcl.Wheel.FR : Subsystem
  CreateBus Vhcl.Wheel.RL : Subsystem
  CreateBus Vhcl.Wheel.RR : Subsystem
  Trailer : S-Function  FunctionName=CM_Sfun  Parameters='Trailer'  EnableBusSupport=off
  Sync_Out : Outport  OutDataType=sfix(16)  OutScaling=2^0
  Vhcl.Steering : Outport  Port=2  OutDataType=sfix(16)  OutScaling=2^0
  Vhcl.Motion : Outport  Port=3  OutDataType=sfix(16)  OutScaling=2^0
  Vhcl.PoI : Outport  Port=4  OutDataType=sfix(16)  OutScaling=2^0
  Vhcl.Wheel.FL : Outport  Port=5  OutDataType=sfix(16)  OutScaling=2^0
  Vhcl.Wheel.FR : Outport  Port=6  OutDataType=sfix(16)  OutScaling=2^0
  Vhcl.Wheel.RL : Outport  Port=7  OutDataType=sfix(16)  OutScaling=2^0
  Vhcl.Wheel.RR : Outport  Port=8  OutDataType=sfix(16)  OutScaling=2^0
  Car.Hitch.FrcTrq : Outport  Port=9  OutDataType=sfix(16)  OutScaling=2^0
  wires:
  Sync_In/1 -> Trailer/1
  Trailer/1 -> Sync_Out/1
  Trailer.Load/1 -> Trailer/2
  Car.Hitch/1 -> Trailer/3
  Car.Fr1/1 -> Trailer/4
  CreateBus Car.Hitch.FrcTrq/1(Car.Hitch.FrcTrq) -> Car.Hitch.FrcTrq/1
  WheelCarrier.Misc/1 -> Trailer/6
  Car.Trq_T2W/1 -> Trailer/5
  CreateBus Vhcl.Motion/1(Out1) -> Vhcl.Motion/1
  CreateBus Vhcl.PoI/1(Out1) -> Vhcl.PoI/1
  CreateBus Vhcl.Wheel.FL/1(Out1) -> Vhcl.Wheel.FL/1  "Vhcl.Wheel.FL"
  CreateBus Vhcl.Wheel.FR/1(Out1) -> Vhcl.Wheel.FR/1  "Vhcl.Wheel.FR"
  CreateBus Vhcl.Wheel.RL/1(Out1) -> Vhcl.Wheel.RL/1  "Vhcl.Wheel.RL"
  CreateBus Vhcl.Wheel.RR/1(Out1) -> Vhcl.Wheel.RR/1  "Vhcl.Wheel.RR"
  Trailer/8 -> CreateBus Vhcl.Wheel.RR/1(In1)
  Trailer/9 -> CreateBus Car.Hitch.FrcTrq/1(In1)
  Trailer/7 -> CreateBus Vhcl.Wheel.RL/1(In1)
  Trailer/6 -> CreateBus Vhcl.Wheel.FR/1(In1)
  Trailer/5 -> CreateBus Vhcl.Wheel.FL/1(In1)
  Trailer/4 -> CreateBus Vhcl.PoI/1(In1)
  Trailer/3 -> CreateBus Vhcl.Motion/1(In1)
  CreateBus Vhcl.Steering/1(Out1) -> Vhcl.Steering/1
  Trailer/2 -> CreateBus Vhcl.Steering/1(In1)

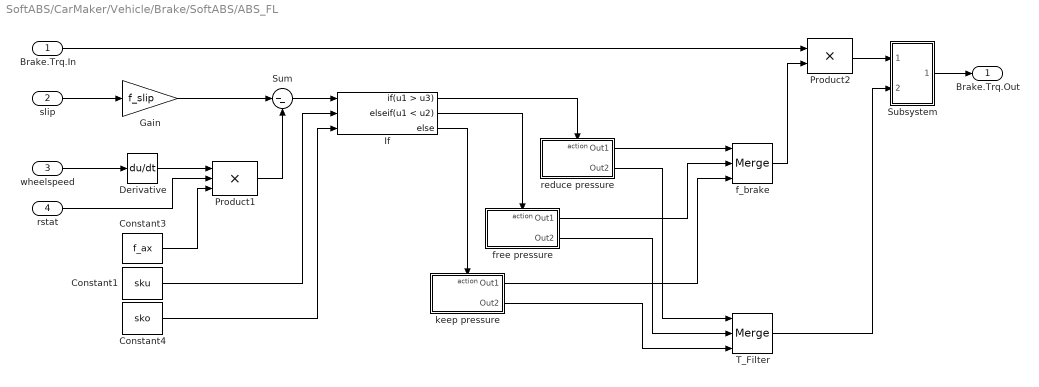
== system SoftABS/CarMaker/Vehicle/Brake/SoftABS/ABS_FL ==
  Brake.Trq.In : Inport  OutDataType=sfix(16)  OutScaling=2^0
  slip : Inport  Port=2  OutDataType=sfix(16)  OutScaling=2^0
  wheelspeed : Inport  Port=3  OutDataType=sfix(16)  OutScaling=2^0
  rstat : Inport  Port=4  OutDataType=sfix(16)  OutScaling=2^0
  Constant1 : Constant  Value=sku  OutDataType=sfix(16)  OutScaling=2^0
  Constant3 : Constant  Value=f_ax  OutDataType=sfix(16)  OutScaling=2^0
  Constant4 : Constant  Value=sko  OutDataType=sfix(16)  OutScaling=2^0
  Derivative : Derivative
  Gain : Gain  Gain=f_slip  ParameterDataType=sfix(16)  ParameterScaling=2^0  OutDataType=sfix(16)  OutScaling=2^0  SaturateOnIntegerOverflow=on  OutDataTypeStr=Inherit: Same as input  ParamDataTypeStr=Inherit: Same as input
  If : If  NumInputs=3  IfExpression=u1 > u3  ElseIfExpressions=u1 < u2
  Product1 : Product  Inputs=3  OutDataType=sfix(16)  OutScaling=2^0  SaturateOnIntegerOverflow=on  InputSameDT=on  OutDataTypeStr=Inherit: Same as first input
  Product2 : Product  OutDataType=sfix(16)  OutScaling=2^0  SaturateOnIntegerOverflow=on  InputSameDT=on  OutDataTypeStr=Inherit: Same as first input
  Subsystem : Subsystem
  Sum : Sum  Inputs=|--  OutDataType=sfix(16)  OutScaling=2^0  SaturateOnIntegerOverflow=on  InputSameDT=on  OutDataTypeStr=Inherit: Same as first input
  T_Filter : Merge  Inputs=3
  f_brake : Merge  Inputs=3
  free pressure : Subsystem  TreatAsAtomicUnit=on
  keep pressure : Subsystem  TreatAsAtomicUnit=on
  reduce pressure : Subsystem  TreatAsAtomicUnit=on
  Brake.Trq.Out : Outport  OutDataType=sfix(16)  OutScaling=2^0
  wires:
  Brake.Trq.In/1 -> Product2/1
  If/3 -> keep pressure/Action
  If/1 -> reduce pressure/Action
  If/2 -> free pressure/Action
  reduce pressure/1(Out1) -> f_brake/1
  free pressure/1(Out1) -> f_brake/2
  keep pressure/1(Out1) -> f_brake/3
  Derivative/1 -> Product1/1
  Gain/1 -> Sum/1
  Product1/1 -> Sum/2
  Sum/1 -> If/1
  slip/1 -> Gain/1
  wheelspeed/1 -> Derivative/1
  rstat/1 -> Product1/2
  reduce pressure/2(Out2) -> T_Filter/1
  free pressure/2(Out2) -> T_Filter/2
  keep pressure/2(Out2) -> T_Filter/3
  f_brake/1 -> Product2/2
  Product2/1 -> Subsystem/1(InFilter)
  Subsystem/1(OutFilter) -> Brake.Trq.Out/1
  T_Filter/1 -> Subsystem/2(TFilter)
  Constant3/1 -> Product1/3
  Constant1/1 -> If/2
  Constant4/1 -> If/3

== system SoftABS/CarMaker/Vehicle/Brake/SoftABS/ABS_FR ==
  Brake.Trq.In : Inport  OutDataType=sfix(16)  OutScaling=2^0
  slip : Inport  Port=2  OutDataType=sfix(16)  OutScaling=2^0
  wheelspeed : Inport  Port=3  OutDataType=sfix(16)  OutScaling=2^0
  rstat : Inport  Port=4  OutDataType=sfix(16)  OutScaling=2^0
  Constant1 : Constant  Value=sku  OutDataType=sfix(16)  OutScaling=2^0
  Constant3 : Constant  Value=f_ax  OutDataType=sfix(16)  OutScaling=2^0
  Constant4 : Constant  Value=sko  OutDataType=sfix(16)  OutScaling=2^0
  Derivative : Derivative
  Gain : Gain  Gain=f_slip  ParameterDataType=sfix(16)  ParameterScaling=2^0  OutDataType=sfix(16)  OutScaling=2^0  SaturateOnIntegerOverflow=on  OutDataTypeStr=Inherit: Same as input  ParamDataTypeStr=Inherit: Same as input
  If : If  NumInputs=3  IfExpression=u1 > u3  ElseIfExpressions=u1 < u2
  Product1 : Product  Inputs=3  OutDataType=sfix(16)  OutScaling=2^0  SaturateOnIntegerOverflow=on  InputSameDT=on  OutDataTypeStr=Inherit: Same as first input
  Product2 : Product  OutDataType=sfix(16)  OutScaling=2^0  SaturateOnIntegerOverflow=on  InputSameDT=on  OutDataTypeStr=Inherit: Same as first input
  Subsystem : Subsystem
  Sum : Sum  Inputs=|--  OutDataType=sfix(16)  OutScaling=2^0  SaturateOnIntegerOverflow=on  InputSameDT=on  OutDataTypeStr=Inherit: Same as first input
  T_Filter : Merge  Inputs=3
  f_brake : Merge  Inputs=3
  free pressure : Subsystem  TreatAsAtomicUnit=on
  keep pressure : Subsystem  TreatAsAtomicUnit=on
  reduce pressure : Subsystem  TreatAsAtomicUnit=on
  Brake.Trq.Out : Outport  OutDataType=sfix(16)  OutScaling=2^0
  wires:
  Brake.Trq.In/1 -> Product2/1
  If/3 -> keep pressure/Action
  If/1 -> reduce pressure/Action
  If/2 -> free pressure/Action
  reduce pressure/1(Out1) -> f_brake/1
  free pressure/1(Out1) -> f_brake/2
  keep pressure/1(Out1) -> f_brake/3
  Derivative/1 -> Product1/1
  Gain/1 -> Sum/1
  Product1/1 -> Sum/2
  Sum/1 -> If/1
  slip/1 -> Gain/1
  wheelspeed/1 -> Derivative/1
  rstat/1 -> Product1/2
  reduce pressure/2(Out2) -> T_Filter/1
  free pressure/2(Out2) -> T_Filter/2
  keep pressure/2(Out2) -> T_Filter/3
  f_brake/1 -> Product2/2
  Product2/1 -> Subsystem/1(InFilter)
  Subsystem/1(OutFilter) -> Brake.Trq.Out/1
  T_Filter/1 -> Subsystem/2(TFilter)
  Constant3/1 -> Product1/3
  Constant1/1 -> If/2
  Constant4/1 -> If/3

== system SoftABS/CarMaker/Vehicle/Brake/SoftABS/ABS_RL ==
  Brake.Trq.In : Inport  OutDataType=sfix(16)  OutScaling=2^0
  slip : Inport  Port=2  OutDataType=sfix(16)  OutScaling=2^0
  wheelspeed : Inport  Port=3  OutDataType=sfix(16)  OutScaling=2^0
  rstat : Inport  Port=4  OutDataType=sfix(16)  OutScaling=2^0
  Constant1 : Constant  Value=sku  OutDataType=sfix(16)  OutScaling=2^0
  Constant3 : Constant  Value=f_ax  OutDataType=sfix(16)  OutScaling=2^0
  Constant4 : Constant  Value=sko  OutDataType=sfix(16)  OutScaling=2^0
  Derivative : Derivative
  Gain : Gain  Gain=f_slip  ParameterDataType=sfix(16)  ParameterScaling=2^0  OutDataType=sfix(16)  OutScaling=2^0  SaturateOnIntegerOverflow=on  OutDataTypeStr=Inherit: Same as input  ParamDataTypeStr=Inherit: Same as input
  If : If  NumInputs=3  IfExpression=u1 > u3  ElseIfExpressions=u1 < u2
  Product1 : Product  Inputs=3  OutDataType=sfix(16)  OutScaling=2^0  SaturateOnIntegerOverflow=on  InputSameDT=on  OutDataTypeStr=Inherit: Same as first input
  Product2 : Product  OutDataType=sfix(16)  OutScaling=2^0  SaturateOnIntegerOverflow=on  InputSameDT=on  OutDataTypeStr=Inherit: Same as first input
  Subsystem : Subsystem
  Sum : Sum  Inputs=|--  OutDataType=sfix(16)  OutScaling=2^0  SaturateOnIntegerOverflow=on  InputSameDT=on  OutDataTypeStr=Inherit: Same as first input
  T_Filter : Merge  Inputs=3
  f_brake : Merge  Inputs=3
  free pressure : Subsystem  TreatAsAtomicUnit=on
  keep pressure : Subsystem  TreatAsAtomicUnit=on
  reduce pressure : Subsystem  TreatAsAtomicUnit=on
  Brake.Trq.Out : Outport  OutDataType=sfix(16)  OutScaling=2^0
  wires:
  Brake.Trq.In/1 -> Product2/1
  If/3 -> keep pressure/Action
  If/1 -> reduce pressure/Action
  If/2 -> free pressure/Action
  reduce pressure/1(Out1) -> f_brake/1
  free pressure/1(Out1) -> f_brake/2
  keep pressure/1(Out1) -> f_brake/3
  Derivative/1 -> Product1/1
  Gain/1 -> Sum/1
  Product1/1 -> Sum/2
  Sum/1 -> If/1
  slip/1 -> Gain/1
  wheelspeed/1 -> Derivative/1
  rstat/1 -> Product1/2
  reduce pressure/2(Out2) -> T_Filter/1
  free pressure/2(Out2) -> T_Filter/2
  keep pressure/2(Out2) -> T_Filter/3
  f_brake/1 -> Product2/2
  Product2/1 -> Subsystem/1(InFilter)
  Subsystem/1(OutFilter) -> Brake.Trq.Out/1
  T_Filter/1 -> Subsystem/2(TFilter)
  Constant3/1 -> Product1/3
  Constant1/1 -> If/2
  Constant4/1 -> If/3

== system SoftABS/CarMaker/Vehicle/Brake/SoftABS/ABS_RR ==
  Brake.Trq.In : Inport  OutDataType=sfix(16)  OutScaling=2^0
  slip : Inport  Port=2  OutDataType=sfix(16)  OutScaling=2^0
  wheelspeed : Inport  Port=3  OutDataType=sfix(16)  OutScaling=2^0
  rstat : Inport  Port=4  OutDataType=sfix(16)  OutScaling=2^0
  Constant1 : Constant  Value=sku  OutDataType=sfix(16)  OutScaling=2^0
  Constant3 : Constant  Value=f_ax  OutDataType=sfix(16)  OutScaling=2^0
  Constant4 : Constant  Value=sko  OutDataType=sfix(16)  OutScaling=2^0
  Derivative : Derivative
  Gain : Gain  Gain=f_slip  ParameterDataType=sfix(16)  ParameterScaling=2^0  OutDataType=sfix(16)  OutScaling=2^0  SaturateOnIntegerOverflow=on  OutDataTypeStr=Inherit: Same as input  ParamDataTypeStr=Inherit: Same as input
  If : If  NumInputs=3  IfExpression=u1 > u3  ElseIfExpressions=u1 < u2
  Product1 : Product  Inputs=3  OutDataType=sfix(16)  OutScaling=2^0  SaturateOnIntegerOverflow=on  InputSameDT=on  OutDataTypeStr=Inherit: Same as first input
  Product2 : Product  OutDataType=sfix(16)  OutScaling=2^0  SaturateOnIntegerOverflow=on  InputSameDT=on  OutDataTypeStr=Inherit: Same as first input
  Subsystem : Subsystem
  Sum : Sum  Inputs=|--  OutDataType=sfix(16)  OutScaling=2^0  SaturateOnIntegerOverflow=on  InputSameDT=on  OutDataTypeStr=Inherit: Same as first input
  T_Filter : Merge  Inputs=3
  f_brake : Merge  Inputs=3
  free pressure : Subsystem  TreatAsAtomicUnit=on
  keep pressure : Subsystem  TreatAsAtomicUnit=on
  reduce pressure : Subsystem  TreatAsAtomicUnit=on
  Brake.Trq.Out : Outport  OutDataType=sfix(16)  OutScaling=2^0
  wires:
  Brake.Trq.In/1 -> Product2/1
  If/3 -> keep pressure/Action
  If/1 -> reduce pressure/Action
  If/2 -> free pressure/Action
  reduce pressure/1(Out1) -> f_brake/1
  free pressure/1(Out1) -> f_brake/2
  keep pressure/1(Out1) -> f_brake/3
  Derivative/1 -> Product1/1
  Gain/1 -> Sum/1
  Product1/1 -> Sum/2
  Sum/1 -> If/1
  slip/1 -> Gain/1
  wheelspeed/1 -> Derivative/1
  rstat/1 -> Product1/2
  reduce pressure/2(Out2) -> T_Filter/1
  free pressure/2(Out2) -> T_Filter/2
  keep pressure/2(Out2) -> T_Filter/3
  f_brake/1 -> Product2/2
  Product2/1 -> Subsystem/1(InFilter)
  Subsystem/1(OutFilter) -> Brake.Trq.Out/1
  T_Filter/1 -> Subsystem/2(TFilter)
  Constant3/1 -> Product1/3
  Constant1/1 -> If/2
  Constant4/1 -> If/3

== system SoftABS/CarMaker/Vehicle/CarAndTrailer/CarAndTrailerUpd/CreateBus Brake.IF.In ==
  In : Inport
  BusCreator : BusCreator  Inputs=9
  Demux : Demux  Outputs=9
  Out : Outport
  wires:
  In/1 -> Demux/1
  BusCreator/1 -> Out/1
  Demux/1 -> BusCreator/1  "Brake IF T_env"
  Demux/2 -> BusCreator/2  "Brake IF Trq_Reg_max FL"
  Demux/3 -> BusCreator/3  "Brake IF Trq_Reg_max FR"
  Demux/4 -> BusCreator/4  "Brake IF Trq_Reg_max RL"
  Demux/5 -> BusCreator/5  "Brake IF Trq_Reg_max RR"
  Demux/6 -> BusCreator/6  "Brake IF Trq_Reg FL"
  Demux/7 -> BusCreator/7  "Brake IF Trq_Reg FR"
  Demux/8 -> BusCreator/8  "Brake IF Trq_Reg RL"
  Demux/9 -> BusCreator/9  "Brake IF Trq_Reg RR"
